simulink model "Iek1_tmp"  (Simulink 8.3)
settings: Solver=FixedStepDiscrete  StartTime=0.0  StopTime=10000000.0  RelTol=1e-3
settings Model: Creator=scaife  LastModifiedBy=bourbouh  CovSFcnEnable=on  ExtModeAutoUpdateStatusClock=off
settings DataIOCC: SignalLoggingName=sigsOut
settings DebuggingCC: SaveWithParameterizedLinksMsg=none  SignalResolutionControl=TryResolveAllWithWarning  SolverPrmCheckMsg=none  MultiTaskDSMMsg=warning  MultiTaskCondExecSysMsg=none  FrameProcessingCompatibilityMsg=error  StateNameClashWarn=none  StrictBusMsg=None
settings HardwareCC: TargetUnknown=on
settings SFSimCC: SimParseCustomCode=off
settings GRTTargetCC: GeneratePreprocessorConditionals=Use local settings

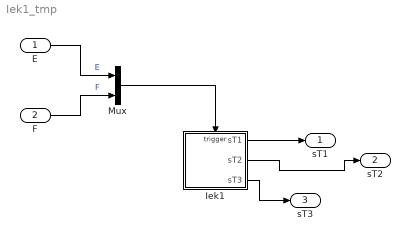
== system Iek1_tmp ==
  E : Inport
  F : Inport  Port=2
  Iek1 : Stateflow chart  TreatAsAtomicUnit=on
      settings: PermitHierarchicalResolution=ParametersOnly
  Mux : Mux  Inputs=2
  sT1 : Outport
  sT2 : Outport  Port=2
  sT3 : Outport  Port=3
  wires:
  F/1 -> Mux/2  "F"
  E/1 -> Mux/1  "E"
  Mux/1 -> Iek1/Trigger
  Iek1/1(sT1) -> sT1/1
  Iek1/2(sT2) -> sT2/1
  Iek1/3(sT3) -> sT3/1

== stateflow chart Iek1 ==
  state T1 [parallel]
    settings: executionOrder=1
    state B
      en: sT1=2
    state A
      en: sT1=1
    (default) -> A
    B -> A : E
    A -> B : E
  state T2 [parallel]
    settings: executionOrder=2
    state C
      en: sT2=1
    state D
      en: sT2=2
    (default) -> C
    D -> C : F
    C -> D : F
  state T3 [parallel]
    settings: executionOrder=3
    state a
      en: sT3=1
    state c
      en: sT3=3
    state b
      en: sT3=2
    state d
      en: sT3=4
    (default) -> a
    a -> c : exit(T1.A)
    b -> c [order 2] : enter(T1.B)
    b -> a [order 1] : enter(T2.C)
    c -> b [order 2] : enter(T2.D)
    c -> d [order 1] : enter(T1.A)
    d -> b : exit(T2.C)
  data: sT1 output double; sT2 output double; sT3 output double
  events: E input EITHER_EDGE_EVENT; F input EITHER_EDGE_EVENT
